simulink model "Problem8"  (R2020b)
settings: Solver=VariableStepAuto  StartTime=0.0  StopTime=10.0  RelTol=1e-3
settings Model: Creator=Shirish  LastModifiedBy=Shirish

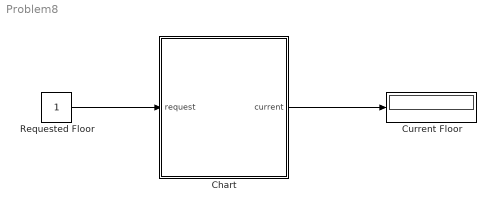
== system Problem8 ==
  Chart : Stateflow chart  TreatAsAtomicUnit=on
  Current Floor : Display
  Requested Floor : Constant
  wires:
  Requested Floor/1 -> Chart/1(request)
  Chart/1(current) -> Current Floor/1

== stateflow chart Problem8/Chart ==
  state Lift
    state Idle
      en: motor=0;
    state Door_closed
      en: door_close=1;
    state Move_Down
      en: motor=-1;
      current=current-1;
    state Move_Up
      en: motor=1;
      current=current+1;
    state Halt
      en: motor=0;
      door_close=1;
    state Door_Open
      door_close=0;
    (default) -> Idle
    Idle -> Idle [order 2] : [request==current]
    Door_Open -> Idle : after(5,sec)
    Idle -> Door_closed [order 1] : after(3,sec)
    Door_closed -> Move_Down [order 2] : [request<current]
    Door_closed -> Move_Up [order 1] : [request>current]
    Move_Up -> Move_Up [order 2] : [request>current]
    Move_Down -> Move_Down [order 2] : [request<current]
    Move_Down -> Halt [order 1] : [request==current]
    Move_Up -> Halt [order 1] : [request==current]
    Halt -> Door_Open : [request==current]
  (default) -> Lift
  data: request input; current output =0; door_close local =0; motor local =0
